simulink model "Wave_based_teleoperation"  (R2019a)
settings: Solver=ode45  StartTime=0.0  StopTime=100  MaxStep=0.01  RelTol=1e-3
undefined symbols (not defined in the file or in its folder): Force
libraries: eeGeneralControl x3, robotlib x3, simulink x2
settings Model: Creator=huic  LastModifiedBy=huic
settings SolverCC: MaxConsecutiveMinStep=1024

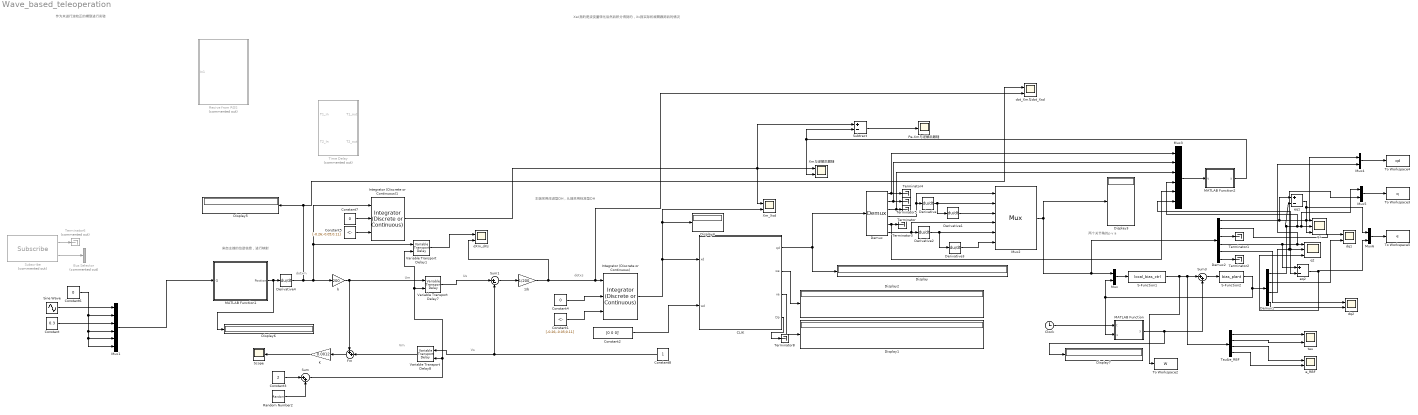
== system Wave_based_teleoperation ==
  note: 作为未进行波校正的模型进行实验
  note: Vm
  note: Us
  note: 主端采用改进型DH，从端采用标准型DH
  note: Vs
  note: dotxs
  note: dotxm
  note: Um
  note: 两个关节角的p v a
  note: Xsd指的是波变量转化后然后积分得到的，Xs指实际机械臂跟踪后的情况
  note: 来自主端的位姿信息，进行映射
  " Time Delay" : Subsystem  Commented=on
  1/b : Gain  Gain=1/200
  Bus Selector : BusSelector  Commented=on  OutputSignals=Position
  CLIK : Subsystem
  Clock : Clock
  Constant : Constant  Value=0.3
  Constant1 : Constant  Value=[-0.26;-0.05;0.11]
  Constant2 : Constant  Value=[0 0 0]'
  Constant3 : Constant  Value=2
  Constant4 : Constant  Value=0
  Constant5 : Constant  Value=[-0.26;-0.05;0.11]
  Constant6 : Constant  Value=0
  Constant7 : Constant  Value=0
  Constant8 : Constant
  Demux : Demux  Outputs=6
  Demux1 : Demux
  Demux2 : Demux  Outputs=6
  Derivative{,1..4} (5 alike) : Derivative
  Display{,1..7} (8 alike) : Display
  Fm : Sum  Inputs=++|
  Integrator (Discrete or Continuous) : eeGeneralControl/Integrator (Discrete or Continuous)  LabelModeActiveChoice=Discrete  ExternalReset=level  LimitType=Anti-windup  B=[0.45;0.45;0.55]  A=[-0.45;-0.45;-0.12]  Ts=-1
      settings: SourceProductName=Simscape Electrical  SourceProductBaseCode=PS
  Integrator (Discrete or Continuous)1 : eeGeneralControl/Integrator (Discrete or Continuous)  LabelModeActiveChoice=Discrete  ExternalReset=level  LimitType=Anti-windup  B=[0.45;0.45;0.55]  A=[-0.45;-0.45;-0.12]  Ts=-1
      settings: SourceProductName=Simscape Electrical  SourceProductBaseCode=PS
  K : Gain  Gain=0.0012
  MATLAB Function : MATLAB Function  TreatAsAtomicUnit=on
  MATLAB Function1 : MATLAB Function  TreatAsAtomicUnit=on
  MATLAB Function2 : MATLAB Function  TreatAsAtomicUnit=on
  Mux{,4..6} (4 alike) : Mux  Inputs=2
  Mux1 : Mux  Inputs=6
  Mux2 : Mux  Inputs=6
  Mux3 : Mux  Inputs=6
  Pe-Xm与逆解后跟随 : Scope
  Random Number2 : RandomNumber  Variance=0.01  SampleTime=0.5
  Recive from ROS : Subsystem  Commented=on
  S-Function1 : S-Function  FunctionName=local_bias_ctrl  SFunctionDeploymentMode=off  EnableBusSupport=off
  S-Function2 : S-Function  FunctionName=bias_plant  SFunctionDeploymentMode=off  EnableBusSupport=off
  Scope : Scope
  Sine Wave : Sin  Amplitude=0.8  Frequency=0.5  SampleTime=0
  Subscribe : robotlib/Subscribe  Commented=on  topicSource=Select from ROS network  topic=/phantom/phantom/joint_states  messageType=sensor_msgs/JointState  sampleTime=-1  messageQueueLength=1
      settings: SourceProductBaseCode=RO
  Subtract : Sum  Inputs=+-
  Sum : Sum  Inputs=|++
  Sum1 : Sum  Inputs=|+-
  Sum3 : Sum  Inputs=|++
  Tau&e_RBF : Demux
  Terminator{,1..5,8} (7 alike) : Terminator
  Terminator6 : Terminator  Commented=on
  To Workspace2 : ToWorkspace  VariableName=W  SaveFormat=Timeseries  SampleTime=-1
  To Workspace3 : ToWorkspace  VariableName=q  SaveFormat=Structure With Time  SampleTime=-1
  To Workspace4 : ToWorkspace  VariableName=qd  SaveFormat=Structure With Time  SampleTime=-1
  To Workspace5 : ToWorkspace  VariableName=e  SaveFormat=Structure With Time  SampleTime=-1
  Variable Transport Delay1 : VariableTransportDelay  MaximumDelay=10  MaximumPoints=10240  ZeroDelay=on
  Variable Transport Delay7 : VariableTransportDelay  MaximumDelay=10  MaximumPoints=10240  ZeroDelay=on
  Variable Transport Delay8 : VariableTransportDelay  MaximumDelay=10  MaximumPoints=10240  ZeroDelay=on
  Xm_Xsd : Scope  NumInputPorts=2
  Xm与逆解后跟随 : Scope  NumInputPorts=2
  b : Gain  Gain=200
  dXm_dXs : Scope  NumInputPorts=2
  dot_Xm与dot_Xsd : Scope  NumInputPorts=2
  dq1 : Scope  NumInputPorts=2
  dq2 : Scope  NumInputPorts=2
  e_RBF : Scope  NumInputPorts=2
  eq1 : Sum  Inputs=+-
  eq2 : Sum  Inputs=+-
  q1 : Scope  NumInputPorts=3
  q2 : Scope  NumInputPorts=3
  tau : Scope  NumInputPorts=2
  wires:
  Mux6/1 -> To Workspace5/1
  Constant1/1 -> Integrator (Discrete or Continuous)/3
  Demux/6 -> Mux2/4, Derivative2/1
  Integrator (Discrete or Continuous)1/1 -> Xm与逆解后跟随/1, Subtract/1, Xm_Xsd/1
  S-Function2/1 -> Demux1/1, MATLAB Function/2(x), Mux/2
  Demux/3 -> Mux3/3, Terminator/1
  Constant6/1 -> Mux1/6, Mux1/5, Mux1/4, Mux1/2
  Mux5/1 -> To Workspace3/1
  Derivative/1 -> Derivative1/1, Mux2/2
  Constant5/1 -> Integrator (Discrete or Continuous)1/3
  Clock/1 -> MATLAB Function/1(t)
  Demux/2 -> Mux3/2, Terminator5/1
  Sine Wave/1 -> Mux1/1
  CLIK/4(Dp) -> Terminator8/1
  MATLAB Function1/1(Postion) -> Display6/1, Derivative4/1
  Mux/1 -> S-Function1/1
  Constant2/1 -> CLIK/2(wd)
  S-Function1/1 -> To Workspace2/1, Sum3/1, Tau&e_RBF/1
  Tau&e_RBF/3 -> e_RBF/1
  Mux4/1 -> To Workspace4/1
  eq2/1 -> Mux6/2, q2/3
  1/b/1 -> dXm_dXs/2, dot_Xm与dot_Xsd/2, Integrator (Discrete or Continuous)/1
  Subtract/1 -> Pe-Xm与逆解后跟随/1
  Demux/5 -> Mux3/5, Terminator3/1
  Demux/4 -> Mux2/1, Derivative/1
  MATLAB Function2/1(y) -> Xm与逆解后跟随/2, Subtract/2
  Demux/1 -> Mux3/1, Terminator4/1
  CLIK/1(qd) -> Display/1, Demux/1
  Sum3/1 -> S-Function2/1
  Sum1/1 -> 1/b/1
  Constant4/1 -> Integrator (Discrete or Continuous)/2
  Constant7/1 -> Integrator (Discrete or Continuous)1/2
  Derivative4/1 -> Variable Transport Delay1/1, Integrator (Discrete or Continuous)1/1, b/1, dot_Xm与dot_Xsd/1, Display5/1
  Demux2/3 -> Terminator1/1
  Constant/1 -> Mux1/3
  Mux3/1 -> MATLAB Function2/1(u)
  Integrator (Discrete or Continuous)/1 -> Display4/1, Xm_Xsd/2, CLIK/1(xd)
  Demux2/5 -> dq2/1
  Tau&e_RBF/2 -> tau/2
  Derivative2/1 -> Derivative3/1, Mux2/5
  Demux1/3 -> q2/2, Mux3/6, eq2/2, Mux5/2
  eq1/1 -> Mux6/1, q1/3
  Tau&e_RBF/1 -> tau/1
  Demux1/2 -> dq1/2
  Demux1/4 -> dq2/2
  Demux2/6 -> Terminator2/1
  Derivative3/1 -> Mux2/6
  Derivative1/1 -> Mux2/3
  Mux2/1 -> Demux2/1, Mux/1, Display3/1
  MATLAB Function/1(y) -> Display7/1, Sum3/2
  CLIK/3(xe) -> Display1/1
  Demux1/1 -> eq1/2, Mux3/4, Mux5/1, q1/2
  Tau&e_RBF/4 -> e_RBF/2
  Demux2/1 -> eq1/1, Mux4/1, q1/1
  CLIK/2(we) -> Display2/1
  Demux2/4 -> Mux4/2, q2/1, eq2/1
  Demux2/2 -> dq1/1
  Subscribe/2 -> Bus Selector/1
  Subscribe/1 -> Terminator6/1
  Mux1/1 -> MATLAB Function1/1(Q)
  Variable Transport Delay8/1 -> Fm/2
  b/1 -> Fm/1, Variable Transport Delay7/1
  Variable Transport Delay7/1 -> Sum1/1
  Constant8/1 -> Sum1/2, Variable Transport Delay8/1
  K/1 -> Scope/1
  Fm/1 -> K/1
  Variable Transport Delay1/1 -> dXm_dXs/1
  Constant3/1 -> Sum/1
  Sum/1 -> Variable Transport Delay1/2, Variable Transport Delay7/2, Variable Transport Delay8/2
  Random Number2/1 -> Sum/2

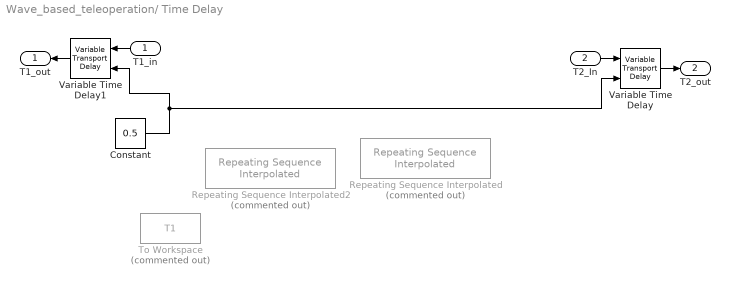
== system Wave_based_teleoperation/ Time Delay ==
  T1_in : Inport
  T2_In : Inport  Port=2
  Constant : Constant  Value=0.5
  Repeating Sequence Interpolated : simulink/Sources/Repeating Sequence Interpolated  Commented=on  OutValues=[0 0 0.21 0.23 0.03 0.03 0.215 0.235 0.03].'  TimeValues=[0 2 4 8 10 12 14 18 20].'  LookUpMeth=Interpolation-Use End Values  tsamp=0.01  OutMin=[]  OutMax=[]  OutDataTypeStr=double  OutputDataTypeScalingMode=double  OutDataType=fixdt(0,8)  OutScaling=2^-10
  Repeating Sequence Interpolated2 : simulink/Sources/Repeating Sequence Interpolated  Commented=on  OutValues=[0 0 0.5 0.52 0.03 0].'  TimeValues=[0 2 4 8 9.8 10].'  LookUpMeth=Interpolation-Use End Values  tsamp=0.01  OutMin=[]  OutMax=[]  OutDataTypeStr=double  OutputDataTypeScalingMode=double  OutDataType=fixdt(0,8)  OutScaling=2^-10
  To Workspace : ToWorkspace  Commented=on  VariableName=T1  SaveFormat=Structure With Time  SampleTime=-1
  Variable Time Delay : VariableTransportDelay  MaximumDelay=10  MaximumPoints=10240  ZeroDelay=on
  Variable Time Delay1 : VariableTransportDelay  MaximumDelay=10  MaximumPoints=10240  ZeroDelay=on
  T1_out : Outport
  T2_out : Outport  Port=2
  wires:
  T1_in/1 -> Variable Time Delay1/1
  Variable Time Delay1/1 -> T1_out/1
  Variable Time Delay/1 -> T2_out/1
  T2_In/1 -> Variable Time Delay/1
  Constant/1 -> Variable Time Delay/2, Variable Time Delay1/2

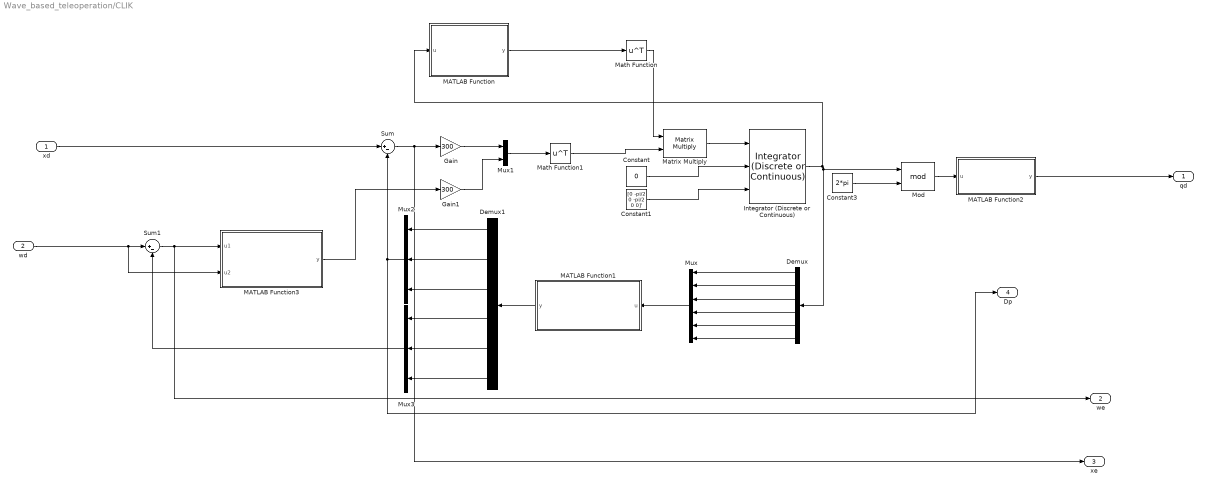
== system Wave_based_teleoperation/CLIK ==
  xd : Inport
  wd : Inport  Port=2
  Constant : Constant  Value=0
  Constant1 : Constant  Value=[0 -pi/2 0 -pi/2 0 0]'
  Constant3 : Constant  Value=2*pi
  Demux : Demux  Outputs=[1 1 1 1 1 1]
  Demux1 : Demux  Outputs=[1 1 1 1 1 1]
  Gain : Gain  Gain=300
  Gain1 : Gain  Gain=300
  Integrator (Discrete or Continuous) : eeGeneralControl/Integrator (Discrete or Continuous)  LabelModeActiveChoice=Continuous  ExternalReset=level  LimitType=Anti-windup  B=inf  A=-inf  Ts=0
      settings: SourceProductName=Simscape Electrical  SourceProductBaseCode=PS
  MATLAB Function : MATLAB Function  TreatAsAtomicUnit=on
  MATLAB Function1 : MATLAB Function  TreatAsAtomicUnit=on
  MATLAB Function2 : MATLAB Function  TreatAsAtomicUnit=on
  MATLAB Function3 : MATLAB Function  TreatAsAtomicUnit=on
  Math Function : Math  Operator=transpose  SaturateOnIntegerOverflow=on
  Math Function1 : Math  Operator=transpose  SaturateOnIntegerOverflow=on
  Matrix Multiply : Product  Multiplication=Matrix(*)
  Mod : Math  Operator=mod  SaturateOnIntegerOverflow=on
  Mux : Mux  Inputs=[1 1 1 1 1 1]
  Mux1 : Mux  Inputs=2
  Mux2 : Mux  Inputs=[1 1 1]
  Mux3 : Mux  Inputs=[1 1 1]
  Sum : Sum  Inputs=|+-
  Sum1 : Sum  Inputs=|+-
  qd : Outport
  we : Outport  Port=2
  xe : Outport  Port=3
  Dp : Outport  Port=4
  wires:
  Demux/2 -> Mux/2
  Gain/1 -> Mux1/1
  Integrator (Discrete or Continuous)/1 -> MATLAB Function/1(u), Demux/1, Mod/1
  Math Function/1 -> Matrix Multiply/1
  Demux/5 -> Mux/5
  Mux/1 -> MATLAB Function1/1(u)
  MATLAB Function2/1(y) -> qd/1
  Mux1/1 -> Math Function1/1
  Demux/4 -> Mux/4
  Demux1/5 -> Mux3/2
  MATLAB Function3/1(y) -> Gain1/1
  Demux/6 -> Mux/6
  wd/1 -> MATLAB Function3/2(u2), Sum1/1
  Demux/1 -> Mux/1
  Demux/3 -> Mux/3
  Matrix Multiply/1 -> Integrator (Discrete or Continuous)/1
  Sum/1 -> xe/1, Gain/1
  Mux3/1 -> Sum1/2
  Constant3/1 -> Mod/2
  Mux2/1 -> Dp/1, Sum/2
  Demux1/4 -> Mux3/1
  Mod/1 -> MATLAB Function2/1(u)
  Demux1/1 -> Mux2/1
  Demux1/2 -> Mux2/2
  Gain1/1 -> Mux1/2
  MATLAB Function1/1(y) -> Demux1/1
  Math Function1/1 -> Matrix Multiply/2
  Demux1/3 -> Mux2/3
  Sum1/1 -> we/1, MATLAB Function3/1(u1)
  Constant1/1 -> Integrator (Discrete or Continuous)/3
  Demux1/6 -> Mux3/3
  xd/1 -> Sum/1
  Constant/1 -> Integrator (Discrete or Continuous)/2
  MATLAB Function/1(y) -> Math Function/1

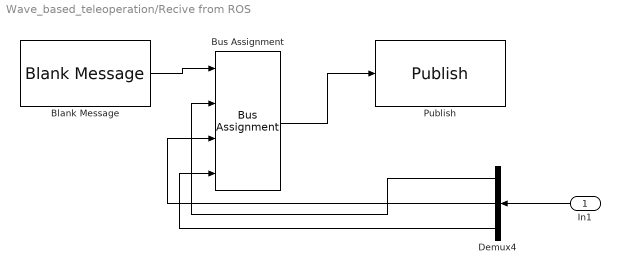
== system Wave_based_teleoperation/Recive from ROS ==
  In1 : Inport
  Blank Message : robotlib/Blank Message  messageClass=Message  entityType=omni_msgs/OmniFeedback  messageType=omni_msgs/OmniFeedback  SampleTime=inf
      settings: SourceProductBaseCode=RO
  Bus Assignment : BusAssignment  AssignedSignals=Force.X,Force.Y,Force.Z
  Demux4 : Demux  Outputs=3
  Publish : robotlib/Publish  topicSource=Select from ROS network  topic=/phantom/phantom/force_feedback  messageType=omni_msgs/OmniFeedback  messageQueueLength=1
      settings: SourceProductBaseCode=RO
  wires:
  In1/1 -> Demux4/1
  Demux4/3 -> Bus Assignment/4
  Demux4/1 -> Bus Assignment/2
  Bus Assignment/1 -> Publish/1
  Demux4/2 -> Bus Assignment/3
  Blank Message/1 -> Bus Assignment/1

== matlab function Wave_based_teleoperation/CLIK/MATLAB Function1 ==
  data: u input; y output
function y = getpose(u)
a2=-0.2035;a3=-0.17442;d1=0.1205;d4=0.08009;
d5=0.08009;d6=0.04436;
q1=u(1);
q2=u(2);
q3=u(3);
q4=u(4);
q5=u(5);
q6=u(6);
%求运动学正解
T01 = [cos(q1) 0 sin(q1) 0;sin(q1) 0 -cos(q1) 0;0 1 0 d1;0 0 0 1];
T12 = [cos(q2) -sin(q2) 0 a2*cos(q2);sin(q2) cos(q2) 0 a2*sin(q2);0 0 1 0;0 0 0 1];
T23 = [cos(q3) -sin(q3) 0 a3*cos(q3);sin(q3) cos(q3) 0 a3*sin(q3);0 0 1 0;0 0 0 1];
T34 = [cos(q4) 0 sin(q4) 0;sin(q4) 0 -cos(q4) 0;0 1 0 d4;0 0 0 1];
T45 = [cos(q5) 0 -sin(q5)  0;sin(q5) 0 cos(q5) 0;0 -1 0 d5;0 0 0 1];
T56 = [cos(q6) -sin(q6) 0 0;sin(q6) cos(q6) 0 0;0 0 1 d6;0 0 0 1];
T06 = T01*T12*T23*T34*T45*T56;

y1=T06(1:3,4);
y2=tform2eul(T06);
y=[y1;y2'];

== matlab function Wave_based_teleoperation/CLIK/MATLAB Function ==
  data: u input; y output
function y = getjacob(u)
%标准型雅可比矩阵求解
a2=-0.2035;a3=-0.17442;d1=0.1205;d4=0.08009;
d5=0.08009;d6=0.04436;
q=u;
%求运动学正解
T01 = [cos(q(1)) 0 sin(q(1)) 0;sin(q(1)) 0 -cos(q(1)) 0;0 1 0 d1;0 0 0 1];
T12 = [cos(q(2)) -sin(q(2)) 0 a2*cos(q(2));sin(q(2)) cos(q(2)) 0 a2*sin(q(2));0 0 1 0;0 0 0 1];
T23 = [cos(q(3)) -sin(q(3)) 0 a3*cos(q(3));sin(q(3)) cos(q(3)) 0 a3*sin(q(3));0 0 1 0;0 0 0 1];
T34 = [cos(q(4)) 0 sin(q(4)) 0;sin(q(4)) 0 -cos(q(4)) 0;0 1 0 d4;0 0 0 1];
T45 = [cos(q(5)) 0 -sin(q(5))  0;sin(q(5)) 0 cos(q(5)) 0;0 -1 0 d5;0 0 0 1];
T56 = [cos(q(6)) -sin(q(6)) 0 0;sin(q(6)) cos(q(6)) 0 0;0 0 1 d6;0 0 0 1];

k = [0; 0; 1];

%初始赋值
Jv = zeros(3, 6);
Jw = zeros(3, 6);
%获取每个关节原点与基座标的变换矩阵T01,T02...T06
% T{6}=zeros(4);
T=cell(6,1);
T{1}=T01;
T{2}=T{1}*T12;
T{3}=T{2}*T23;
T{4}=T{3}*T34;
T{5}=T{4}*T45;
T{6}=T{5}*T56;

%进行矢量积求解
for i = 1: 6
   if i == 1
       R = eye(3);
       p_im = T{6}(1: 3, 4);
   else
       R = T{i-1}(1: 3, 1: 3);
       p_im = T{6}(1: 3, 4) - T{i-1}(1: 3, 4);
   end
   
   zi_1 = R * k;
   Jv(:, i) = cross(zi_1, p_im);
   Jw(:, i) = zi_1;
end

% 组合
J = [Jv; Jw];
y=J;

== matlab function Wave_based_teleoperation/CLIK/MATLAB Function2 ==
  data: u input; y output
function y = Joints_angle_Handle(u)
for i=1:5
    if(u(i) > pi)
        u(i) = u(i)-2*pi;
    elseif(u(i) < -pi)
        u(i) = u(i)+2*pi;
    end
end

y = u;

== matlab function Wave_based_teleoperation/CLIK/MATLAB Function3 ==
  data: u1 input; y output; u2 input
function y = anglevelocity(u1,u2)
%u2为当前的欧拉角
%u1为欧拉角的变化量
tform=[cos(u2(2))*cos(u2(3)) -sin(u2(3)) 0;cos(u2(2))*sin(u2(3)) cos(u2(3)) 0;-sin(u2(2)) 0 1];
y=zeros(1,3);
dwxyz=tform*[u1(3);u1(2);u1(1)];
y(1)=dwxyz(1);
y(2)=dwxyz(2);
y(3)=dwxyz(3);

== matlab function Wave_based_teleoperation/MATLAB Function ==
  data: t input; y output; x input
function y = turbulence(t,x)
Td=zeros(64,1);
if t>30&&t<35
    l1 = 0.35;  %unit is 'm'
    l2 = 0.31;  % li is the length of ith link i
    J=[-l1*sin(x(1))+l2*sin(x(1)+x(3))  -l2*sin(x(1)+x(3));  l1*cos(x(1))+l2*cos(x(1)+x(3))  l2*cos(x(1)+x(3)) ];
%     Td(1:2,:)=J'*[4,8]';
    Td(1:2,:)=J'*[10,16]';
end
y=Td;
end

== matlab function Wave_based_teleoperation/MATLAB Function1 ==
  data: Q input; Postion output
function Postion = TouchX_to_Gluon(Q)
d4=0.13335;d6=0.03;a2=0.13335;
q1=Q(1);q2=Q(2);q3=Q(3);q4=Q(4);q5=Q(5);q6=Q(6);
T01=[cos(q1) -sin(q1) 0 0;sin(q1) cos(q1) 0 0;0 0 1 0;0 0 0 1];
T12=[cos(q2) -sin(q2) 0 0;0 0 -1 0;sin(q2) cos(q2) 0 0;0 0 0 1];
T23=[cos(q3) -sin(q3) 0 a2;sin(q3) cos(q3) 0 0;0 0 1 0;0 0 0 1];
T34=[cos(q4) -sin(q4) 0 0;0 0 -1 -d4;sin(q4) cos(q4) 0 0;0 0 0 1];
T45=[cos(q5) -sin(q5) 0 0;0 0 -1 0;sin(q5) cos(q5) 0 0;0 0 0 1];
T56=[cos(q6) -sin(q6) 0 0;0 0 1 d6;-sin(q6) -cos(q6) 0 0;0 0 0 1];

T06=T01*T12*T23*T34*T45*T56;
%进行映射转换
 Xg = 2.4*T06(1,4)-0.26;
 Yg = 1.6*T06(2,4)-0.05;
 Zg = 1.4*T06(3,4)+0.11;
%进行映射后的笛卡尔空间位置
P=[Xg;Yg;Zg];
% pose=tform2eul(T06);
Postion = P;
% Pose=pose';

== matlab function Wave_based_teleoperation/MATLAB Function2 ==
  data: u input; y output
function y = Position(u)
a2=-0.2035;a3=-0.17442;d1=0.1205;d4=0.08009;
d5=0.08009;
q1=u(1);
q2=u(2);
q3=u(3);
q4=u(4);
q5=u(5);
q6=u(6);
%求运动学正解
T01 = [cos(q1) 0 sin(q1) 0;sin(q1) 0 -cos(q1) 0;0 1 0 d1;0 0 0 1];
T12 = [cos(q2) -sin(q2) 0 a2*cos(q2);sin(q2) cos(q2) 0 a2*sin(q2);0 0 1 0;0 0 0 1];
T23 = [cos(q3) -sin(q3) 0 a3*cos(q3);sin(q3) cos(q3) 0 a3*sin(q3);0 0 1 0;0 0 0 1];
T34 = [cos(q4) 0 sin(q4) 0;sin(q4) 0 -cos(q4) 0;0 1 0 d4;0 0 0 1];
T45 = [cos(q5) 0 -sin(q5)  0;sin(q5) 0 cos(q5) 0;0 -1 0 d5;0 0 0 1];
T56 = [cos(q6) -sin(q6) 0 0;sin(q6) cos(q6) 0 0;0 0 1 0;0 0 0 1];
T06 = T01*T12*T23*T34*T45*T56;

y1=T06(1:3,4);
y=y1;
